simulink model "untitled"  (R2020b)
settings: Solver=VariableStepAuto  StartTime=0.0  StopTime=7200  RelTol=1e-3
settings Model: Creator=Usuario  LastModifiedBy=Usuario
settings ConfigComp: CovScope=Subsystem  CovPath=OBDH

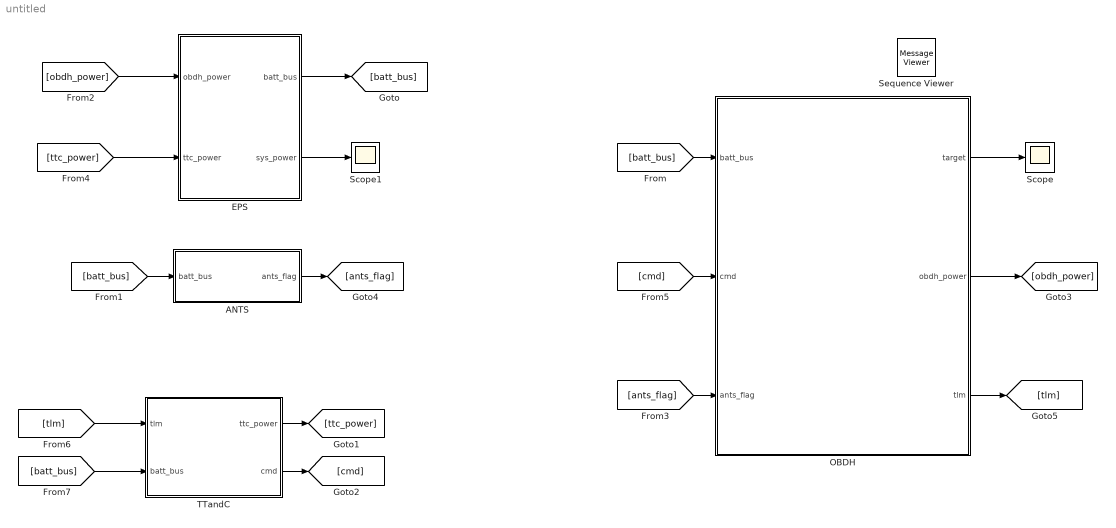
== system untitled ==
  ANTS : Stateflow chart  TreatAsAtomicUnit=on
  EPS : Subsystem
  OBDH : Stateflow chart  TreatAsAtomicUnit=on
  Scope : Scope
  Scope1 : Scope
  Sequence Viewer : MessageViewer  History=1000  SavedRootId=#
  TTandC : Subsystem
  wires:
  [batt_bus] -> OBDH/1(batt_bus)
  [batt_bus] -> ANTS/1(batt_bus)
  [cmd] -> OBDH/2(cmd)
  OBDH/1(target) -> Scope/1
  OBDH/2(obdh_power) -> [obdh_power]
  ANTS/1(ants_flag) -> [ants_flag]
  [ants_flag] -> OBDH/3(ants_flag)
  [obdh_power] -> EPS/1(obdh_power)
  EPS/1(batt_bus) -> [batt_bus]
  EPS/2(sys_power) -> Scope1/1
  [ttc_power] -> EPS/2(ttc_power)
  TTandC/1(ttc_power) -> [ttc_power]
  TTandC/2(cmd) -> [cmd]
  OBDH/3(tlm) -> [tlm]
  [tlm] -> TTandC/1(tlm)
  [batt_bus] -> TTandC/2(batt_bus)

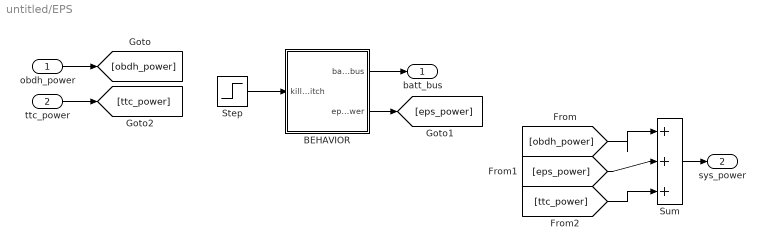
== system untitled/EPS ==
  obdh_power : Inport
  ttc_power : Inport  Port=2
  BEHAVIOR : Stateflow chart  TreatAsAtomicUnit=on
  Step : Step  Time=600  Before=1  After=0  SampleTime=0
  Sum : Sum  Inputs=|+++
  batt_bus : Outport
  sys_power : Outport  Port=2
  wires:
  Sum/1 -> sys_power/1
  BEHAVIOR/1(batt_bus) -> batt_bus/1
  Step/1 -> BEHAVIOR/1(killswitch)
  obdh_power/1 -> [obdh_power]
  [obdh_power] -> Sum/1
  BEHAVIOR/2(eps_power) -> [eps_power]
  [eps_power] -> Sum/2
  ttc_power/1 -> [ttc_power]
  [ttc_power] -> Sum/3

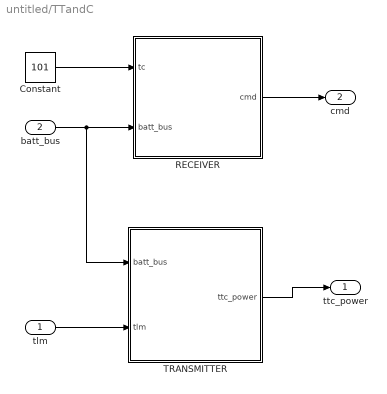
== system untitled/TTandC ==
  tlm : Inport
  batt_bus : Inport  Port=2
  Constant : Constant  Value=101
  RECEIVER : Stateflow chart  TreatAsAtomicUnit=on
  TRANSMITTER : Stateflow chart  TreatAsAtomicUnit=on
      settings: PortSchema="{\"entries\":[{\"content\":{\"sides\":[{\"content\":{\"connectorIds\":[\"In2\",\"In1\"]},\"type\":\"ConnectorPlacement.EquallySpacedRectSide\",\"uuid\":\"6faeabe4-0815-4da5-af70-1287546cbc59\"},{\"content\":{\"connectorIds\":[\"Out1\"],\"side\":\"RIGHT\"},\"type\":\"ConnectorPlacement.EquallySpacedRectSide\",\"uuid\":\"2e787a61-8032-4c93-9bbd-5801bbb92ae3\"},{\"content\":{\"connectorIds\":[],\"side\":\"TOP\"},\"type\":\"ConnectorPlacement.EquallySpacedRectSide\",\"uuid\":\"25a0ca1d-a859-432e-817c-0269a9d3d484\"},{\"content\":{\"connectorIds\":[],\"side\":\"HIDDEN\"},\"type\":\"ConnectorPlacement.EquallySpacedRectSide\",\"uuid\":\"24151c9a-d597-4813-8ea0-ee382c72ce11\"}]},\"type\":\"ConnectorPlacement.EquallySpacedConnector\",\"uuid\":\"302bb981-2935-4333-ad13-3e59b5139db3\"}],\"packageUris\":[\"http://schema.mathworks.com/mf0/Connector/R2020b\"],\"version\":\"1.0\"}"
  ttc_power : Outport
  cmd : Outport  Port=2
  wires:
  tlm/1 -> TRANSMITTER/1(tlm)
  TRANSMITTER/1(ttc_power) -> ttc_power/1
  RECEIVER/1(cmd) -> cmd/1
  Constant/1 -> RECEIVER/1(tc)
  batt_bus/1 -> TRANSMITTER/2(batt_bus), RECEIVER/2(batt_bus)

== stateflow chart untitled/TTandC/RECEIVER ==
  state off
  state on
    state idle
    state receiving
      entry:
      cmd = tc
    (default) -> idle
    idle -> receiving : after(15,sec)
    receiving -> idle : after(5,sec)
  (default) -> off
  on -> off : [batt_bus == 0]
  off -> on : [batt_bus == 1]
  data: tc input; cmd output; batt_bus input

== stateflow chart untitled/TTandC/TRANSMITTER ==
  state off
  state on
    state nominal
      state idle
        entry:
        ttc_power = 1e-6;
      state transmitting
        entry:
        ttc_power = 1e-3;
      (default) -> idle
      idle -> transmitting : [tlm == 1]
      transmitting -> idle : [tlm == 0]
    state emergency
    (default) -> nominal
    (junction 14) -> nominal : [error_flag == 0]
    nominal -> (junction 9) : [error_flag == 1]
    emergency -> (junction 14)
    (junction 9) -> emergency
  (default) -> off
  off -> on : [batt_bus == 1]
  on -> off : [batt_bus == 0]
  data: ttc_power output; tlm input; error_flag local =0; batt_bus input

== stateflow chart untitled/EPS/BEHAVIOR ==
  state on
    entry:
    batt_bus = 1;
    eps_power = 1e-6;
  state off
    entry:
    batt_bus = 0;
    eps_power = 0;
  (default) -> off : {vbatt = 100}
  off -> on : [killswitch == 0]
  (junction 9) -> off
  on -> (junction 9) : [vbatt < 10]
  data: killswitch input; batt_bus output; vbatt local; eps_power output

== stateflow chart untitled/ANTS ==
  state idle
  state burning
  state deployed
    entry:
    ants_flag = 1;
  (default) -> idle
  idle -> burning : [batt_bus == 1]
  burning -> deployed : after(2400,sec)
  data: batt_bus input; ants_flag output

== stateflow chart untitled/OBDH ==
  state on
    state boot
      entry:
      error_ants = 0
    state deployment
      during:
      error_ants = error_ants + 1
    state operational
      state safe
        entry:
        obdh_power = 1e-6;
        target = 0;
        tlm = 1;
      state nominal
        entry:
        tlm = 2;
      (default) -> safe
      safe -> nominal : [cmd == 101]
      nominal -> safe : [cmd == 102]
    (default) -> boot
    boot -> deployment : after(1800,sec)
    (junction 32) -> boot
    deployment -> operational : [ants_flag == 1 || error_ants > 10]
    operational -> (junction 32) : [cmd == 901]
  state off
  (default) -> off : {obdh_power = 0}
  off -> on : [batt_bus == 1]
  (junction 41) -> off
  on -> (junction 41) : [batt_bus == 0]
  data: batt_bus input; cmd input; ants_flag input; error_ants local; target output; obdh_power output; tlm output
